simulink model "impedanceControl"  (Simulink 8.3)
settings: Solver=FixedStepDiscrete  StartTime=0.0  StopTime=simulationTime  FixedStep=Ts  RelTol=1e-3
InitFcn:
  | init_impedanceControl;
values from neighbouring files (symbols this model uses):
  AMPLS = 15*ones(1,ROBOT_DOF)    [init_impedanceControl.m]
  FREQS = 0.25*ones(1,ROBOT_DOF)    [init_impedanceControl.m]
  GRAV_COMP = 1    [init_impedanceControl.m]
  Kd = 2*sqrt(Kp)*0    [init_impedanceControl.m]
  Kp = diag([KpTorso,KpArms,KpArms])    [init_impedanceControl.m]
  MOVING = 0    [init_impedanceControl.m]
  ROBOT_DOF = 11    [init_impedanceControl.m]
libraries: WBCLibrary x14
settings Model: Creator=daniele  LastModifiedBy=daniele
settings DebuggingCC: UnderspecifiedInitializationDetection=Simplified  MergeDetectMultiDrivingBlocksExec=error  MultiTaskDSMMsg=warning  MultiTaskCondExecSysMsg=none  StateNameClashWarn=none  StrictBusMsg=ErrorOnBusTreatedAsVector
settings RTWCC: IncludeERTFirstTime=on
settings GRTTargetCC: CombineOutputUpdateFcns=on  GRTInterface=off

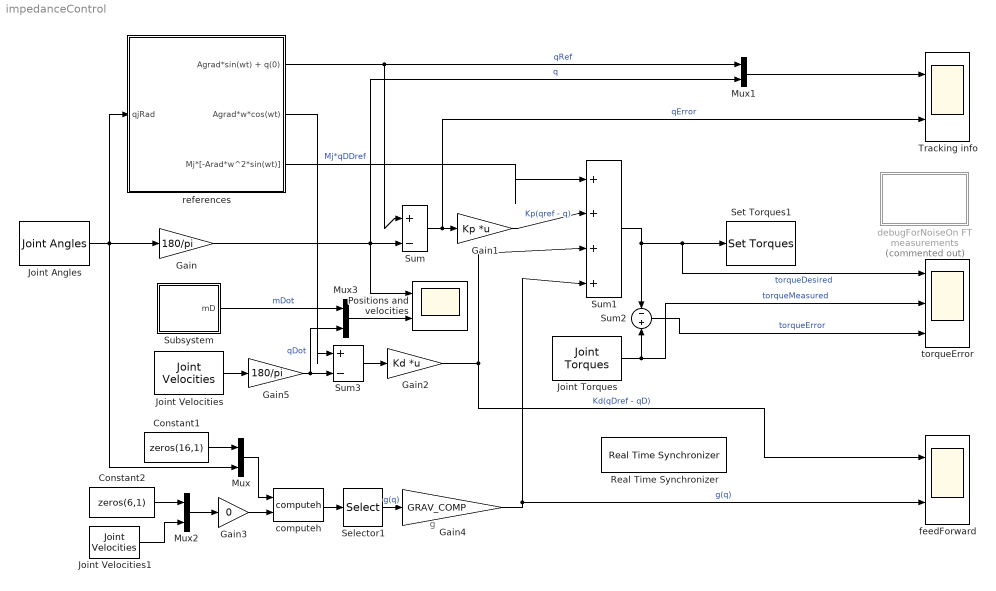
== system impedanceControl ==
  note: g
  Constant1 : Constant  Value=zeros(16,1)
  Constant2 : Constant  Value=zeros(6,1)
  Gain : Gain  Gain=180/pi
  Gain1 : Gain  Gain=Kp  Multiplication=Matrix(K*u)
  Gain2 : Gain  Gain=Kd  Multiplication=Matrix(K*u)
  Gain3 : Gain  Gain=0
  Gain4 : Gain  Gain=GRAV_COMP
  Gain5 : Gain  Gain=180/pi
  Joint Angles : WBCLibrary/wholeBodyStates/Joint Angles  robotName=robotName  localName=localName
  Joint Torques : WBCLibrary/wholeBodyStates/Joint Torques  robotName=robotName  localName=localName
  Joint Velocities : WBCLibrary/wholeBodyStates/Joint Velocities  robotName=robotName  localName=localName
  Joint Velocities1 : WBCLibrary/wholeBodyStates/Joint Velocities  robotName=robotName  localName=localName
  Mux{,1..3} (4 alike) : Mux  Inputs=2
  "Positions and velocities " : Scope  NumInputPorts=2
      settings: ShowLegends=on  TimeRange=10  YMin=8~-30  YMax=20~40  SaveName=ScopeData4
  Real Time Synchronizer : WBCLibrary/Utilities/Real Time Synchronizer  Priority=-10  threadPeriod=Ts
  Selector1 : Selector  InputPortWidth=ROBOT_DOF+6  Indices=[7:ROBOT_DOF+6]
  Set Torques1 : WBCLibrary/wholeBodyActuators/Set Torques  val=6  robotName=robotName  localName=localName
  Subsystem : Subsystem
  Sum : Sum  Inputs=|+-
  Sum1 : Sum  Inputs=|++++
  Sum2 : Sum  Inputs=-|+
  Sum3 : Sum  Inputs=|+-
  Tracking info : Scope  NumInputPorts=2
      settings: ShowLegends=on  TimeRange=20  YMin=-60~-20  YMax=80~15  SaveName=ScopeData3
  computeh : WBCLibrary/wholeBodyModel/Dynamics/computeh  val=7  robotname=robotName  localname=localName
  debugForNoiseOn FT measurements : Subsystem  Commented=on
  feedForward : Scope  NumInputPorts=2
      settings: ShowLegends=on  TimeRange=70  YMin=-5~-5  YMax=4~5
  references : Subsystem
  torqueError : Scope  NumInputPorts=3
      settings: ShowLegends=on  TimeRange=20  YMin=-3~-2~-2  YMax=3~3~2
  wires:
  Gain/1 -> "Positions and velocities "/1, Sum/2, Mux1/2  "q"
  Sum/1 -> Tracking info/2, Gain1/1  "qError"
  Gain1/1 -> Sum1/2  "Kp(qref - q)"
  Joint Velocities/1 -> Gain5/1
  Gain2/1 -> Sum1/3, feedForward/1  "Kd(qDref - qD)"
  Sum1/1 -> Sum2/1, torqueError/1, Set Torques1/1  "torqueDesired"
  Gain3/1 -> computeh/2
  computeh/1 -> Selector1/1
  Mux/1 -> computeh/1
  Joint Angles/1 -> Mux/2, references/1(qjRad), Gain/1
  Constant1/1 -> Mux/1
  Selector1/1 -> Gain4/1  "g(q)"
  Joint Torques/1 -> torqueError/2, Sum2/2  "torqueMeasured"
  Sum2/1 -> torqueError/3  "torqueError"
  Mux2/1 -> Gain3/1
  Constant2/1 -> Mux2/1
  Joint Velocities1/1 -> Mux2/2
  Gain4/1 -> Sum1/4, feedForward/2  "g(q)"
  Mux1/1 -> Tracking info/1
  references/1(Agrad*sin(wt) + q(0)) -> Sum/1, Mux1/1  "qRef"
  Gain5/1 -> Mux3/2, Sum3/2  "qDot"
  Sum3/1 -> Gain2/1
  references/2(Agrad*w*cos(wt)) -> Sum3/1
  references/3(Mj*[-Arad*w^2*sin(wt)]) -> Sum1/1  "Mj*qDDref"
  Mux3/1 -> "Positions and velocities "/2
  Subsystem/1(mD) -> Mux3/1  "mDot"

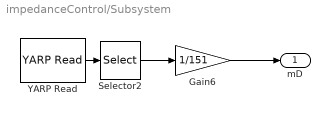
== system impedanceControl/Subsystem ==
  Gain6 : Gain  Gain=1/151
  Selector2 : Selector  InputPortWidth=6  Indices=[1]
  YARP Read : WBCLibrary/Utilities/YARP Read  portName='/controlBoardDumper/right_leg/getMotorEncoderSpeeds'  signalSize=6  blocking=off  timestamp=off  autoconnect=on  errorOnConnection=off
  mD : Outport
  wires:
  YARP Read/1 -> Selector2/1
  Selector2/1 -> Gain6/1
  Gain6/1 -> mD/1

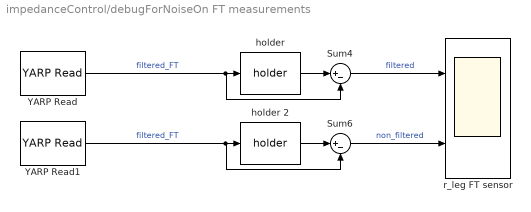
== system impedanceControl/debugForNoiseOn FT measurements ==
  Sum4 : Sum  Inputs=|+-
  Sum6 : Sum  Inputs=|+-
  YARP Read : WBCLibrary/Utilities/YARP Read  portName='/wholeBodyDynamicsTree/filtered/r_leg_ft_sensor:o'  signalSize=6  blocking=off  timestamp=off  autoconnect=on  errorOnConnection=off
  YARP Read1 : WBCLibrary/Utilities/YARP Read  portName='/icub/right_leg/analog:o'  signalSize=6  blocking=off  timestamp=off  autoconnect=on  errorOnConnection=off
  "holder " : WBCLibrary/Utilities/holder 
  holder 2 : WBCLibrary/Utilities/holder 
  r_leg FT sensor : Scope  NumInputPorts=2
      settings: ShowLegends=on  TimeRange=10  YMin=-10~-15  YMax=15~20  SaveName=ScopeData5
  wires:
  "holder "/1 -> Sum4/1
  YARP Read/1 -> Sum4/2, "holder "/1  "filtered_FT"
  Sum6/1 -> r_leg FT sensor/2  "non_filtered"
  YARP Read1/1 -> Sum6/2, holder 2/1  "filtered_FT"
  holder 2/1 -> Sum6/1
  Sum4/1 -> r_leg FT sensor/1  "filtered"

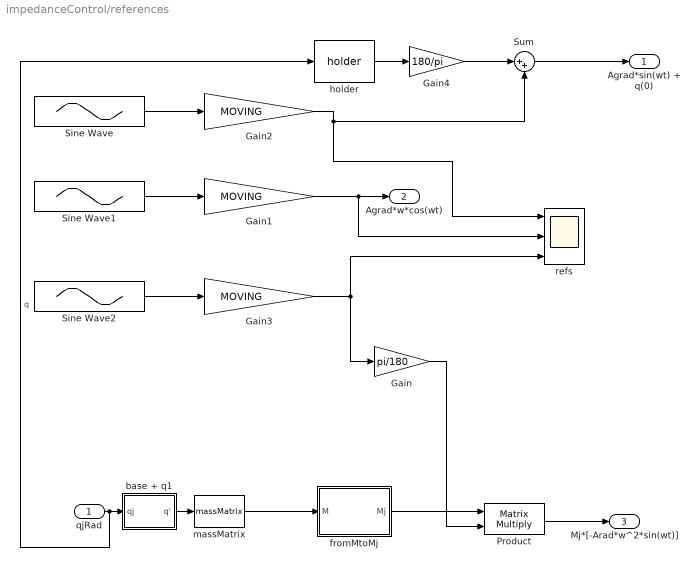
== system impedanceControl/references ==
  qjRad : Inport
  Gain : Gain  Gain=pi/180
  Gain1 : Gain  Gain=MOVING
  Gain2 : Gain  Gain=MOVING
  Gain3 : Gain  Gain=MOVING
  Gain4 : Gain  Gain=180/pi
  Product : Product  Multiplication=Matrix(*)
  Sine Wave : Sin  Amplitude=AMPLS  Frequency=FREQS*2*pi  SampleTime=0
  Sine Wave1 : Sin  Amplitude=AMPLS.*FREQS*2*pi  Frequency=FREQS*2*pi  Phase=pi/2  SampleTime=0
  Sine Wave2 : Sin  Amplitude=-AMPLS.*(FREQS*2*pi).^2  Frequency=FREQS*2*pi  SampleTime=0
  Sum : Sum  Inputs=|++
  base + q1 : Subsystem
  fromMtoMj : MATLAB Function  TreatAsAtomicUnit=on
  "holder " : WBCLibrary/Utilities/holder 
  massMatrix : WBCLibrary/wholeBodyModel/Dynamics/massMatrix  val=8  robotname=robotName  localname=localName
  refs : Scope  NumInputPorts=3
      settings: ShowLegends=on  TimeRange=70  YMin=-5~-5~-5  YMax=4~5~5  SaveName=ScopeData2
  Agrad*sin(wt) + q(0) : Outport
  Agrad*w*cos(wt) : Outport  Port=2
  Mj*[-Arad*w^2*sin(wt)] : Outport  Port=3
  wires:
  Sine Wave/1 -> Gain2/1
  Gain2/1 -> Sum/2, refs/1
  Sine Wave1/1 -> Gain1/1
  Gain1/1 -> refs/2, Agrad*w*cos(wt)/1
  Sine Wave2/1 -> Gain3/1
  base + q1/1(q') -> massMatrix/1
  Product/1 -> Mj*[-Arad*w^2*sin(wt)]/1
  massMatrix/1 -> fromMtoMj/1(M)
  fromMtoMj/1(Mj) -> Product/1
  Gain3/1 -> Gain/1, refs/3
  Gain/1 -> Product/2
  qjRad/1 -> "holder "/1, base + q1/1(qj)  "q"
  Sum/1 -> Agrad*sin(wt) + q(0)/1
  "holder "/1 -> Gain4/1
  Gain4/1 -> Sum/1

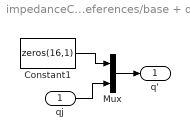
== system impedanceControl/references/base + q1 ==
  qj : Inport
  Constant1 : Constant  Value=zeros(16,1)
  Mux : Mux  Inputs=2
  q' : Outport
  wires:
  Mux/1 -> q'/1
  qj/1 -> Mux/2
  Constant1/1 -> Mux/1

== matlab function references/fromMtoMj ==
  data: M input double; Mj output double
function Mj = fromMtoMj(M)
%#codegen

Mj = M(7:end,7:end);
